simulink model "factorial_whileLoop"  (R2021a)
settings: Solver=FixedStepAuto  StartTime=0.0  StopTime=10.0  RelTol=1e-3
settings Model: Creator=user  LastModifiedBy=user
settings OptimizationCC: DefaultParameterBehavior=Inlined  EnhancedBackFolding=on  PassReuseOutputArgsAs=Individual arguments  ZeroExternalMemoryAtStartup=off  ZeroInternalMemoryAtStartup=off  OptimizeBlockOrder=speed  DifferentSizesBufferReuse=on  OptimizationCustomize=off  EfficientTunableParamExpr=on
settings DebuggingCC: ParameterTunabilityLossMsg=error
settings SFSimCC: MATLABDynamicMemAlloc=off
settings RTWCC: SystemTargetFile=ert.tlc  GenCodeOnly=on  TemplateMakefile=ert_default_tmf  GenerateReport=on  IncludeHyperlinkInReport=on  LaunchReport=on  GenerateTraceInfo=on
settings CodeAppCC: ForceParamTrailComments=on  IgnoreCustomStorageClasses=off  OperatorAnnotations=on  SimulinkDataObjDesc=on  SFDataObjDesc=on  InsertBlockDesc=on
settings ERTTargetCC: TargetLangStandard=C99 (ISO)  GenerateSampleERTMain=on  InlinedParameterPlacement=NonHierarchical  ERTCustomFileTemplate=example_file_process.tlc

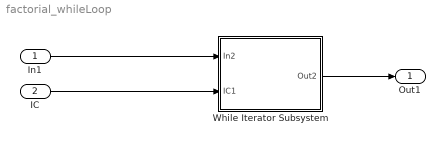
== system factorial_whileLoop ==
  In1 : Inport
  IC : Inport  Port=2
  While Iterator Subsystem : Subsystem  TreatAsAtomicUnit=on
  Out1 : Outport
  wires:
  While Iterator Subsystem/1(Out2) -> Out1/1
  In1/1 -> While Iterator Subsystem/1(In2)
  IC/1 -> While Iterator Subsystem/2(IC1)

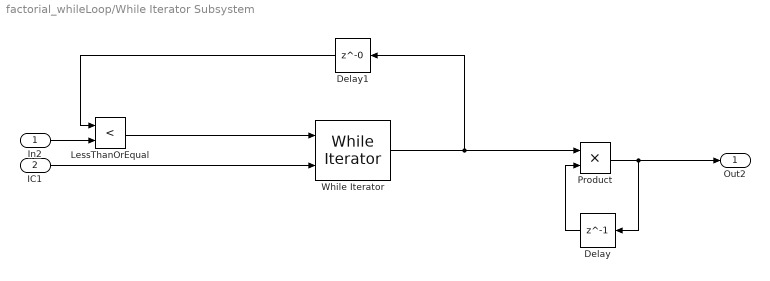
== system factorial_whileLoop/While Iterator Subsystem ==
  In2 : Inport
  IC1 : Inport  Port=2
  Delay : Delay  DelayLength=1  InitialCondition=1
  Delay1 : Delay  DelayLength=0  InitialCondition=0
  LessThanOrEqual : RelationalOperator  Operator=<  OutDataTypeStr=boolean  RndMeth=Simplest
  Product : Product  OutDataTypeStr=int32
  While Iterator : WhileIterator  MaxIters=-1  ShowIterationPort=on
  Out2 : Outport
  wires:
  LessThanOrEqual/1 -> While Iterator/1
  IC1/1 -> While Iterator/2
  In2/1 -> LessThanOrEqual/2
  Delay1/1 -> LessThanOrEqual/1
  Product/1 -> Out2/1, Delay/1
  Delay/1 -> Product/2
  While Iterator/1 -> Delay1/1, Product/1
